simulink model "wheat_line_20_travelling_wind_2019b"  (R2019b)
settings: Solver=FixedStepAuto  StartTime=0.0  StopTime=20  FixedStep=0.001  RelTol=1e-3
values from neighbouring files (symbols this model uses):
  alpha = 50    [run_wheat_line_sway_experiment.m]
  beta = 0    [run_wheat_line_sway_experiment.m]
  edge = 0.1    [natural_freq_experiment.m]    (also in run_wheat_field_sine_wind.m; run_wheat_field_sine_wind_random_height.m; run_wheat_line_experiment.m; run_wheat_line_sway_experiment.m)
  field_length = 4    [natural_freq_experiment.m]    (also in run_wheat_field_sine_wind.m; run_wheat_field_sine_wind_random_height.m; run_wheat_line_experiment.m; run_wheat_line_sway_experiment.m = 8)
  force_amplitude = 5    [natural_freq_experiment.m]    (also in run_wheat_line_sway_experiment.m)
  gain = -800    [natural_freq_experiment.m]    (also in run_wheat_line_experiment.m; run_wheat_line_sway_experiment.m; set_wheat_params.m)
  if_wind_sine = 0    [run_wheat_line_sway_experiment.m]
  wheat_gap = wheat_stem_height/2    (= 0.4)    [natural_freq_experiment.m]    (also in run_wheat_field_sine_wind.m; run_wheat_field_sine_wind_random_height.m; run_wheat_line_experiment.m; run_wheat_line_sway_experiment.m)
  wheat_grain_height = 0.15    [natural_freq_experiment.m]    (also in run_wheat_field_sine_wind.m; run_wheat_field_sine_wind_random_height.m; run_wheat_line_experiment.m; run_wheat_line_sway_experiment.m)
  wheat_grain_radius = 0.03    [natural_freq_experiment.m]    (also in run_wheat_field_sine_wind.m; run_wheat_field_sine_wind_random_height.m; run_wheat_line_experiment.m; run_wheat_line_sway_experiment.m)
  wind_amplitude = 1    [create_travelling_wind_rectangle.m]    (also in create_travelling_wind_sine.m; run_wheat_line_sway_experiment.m)
  wind_frequency = 2    [create_travelling_wind_rectangle.m]    (also in create_travelling_wind_sine.m = 5; run_wheat_line_sway_experiment.m = 50)
  wind_phase_cycle = 5    [create_travelling_wind_rectangle.m]    (also in create_travelling_wind_sine.m = 10; run_wheat_line_sway_experiment.m = 250)
undefined symbols (not defined in the file or in its folder): force_frequency, X, Y, Z
libraries: sm_lib x145, nesl_utility x101, dspmtrx3 x2, dspindex x2, simulink x2
(part 1 of 11)
settings Model: Creator=yz655  LastModifiedBy=Emily

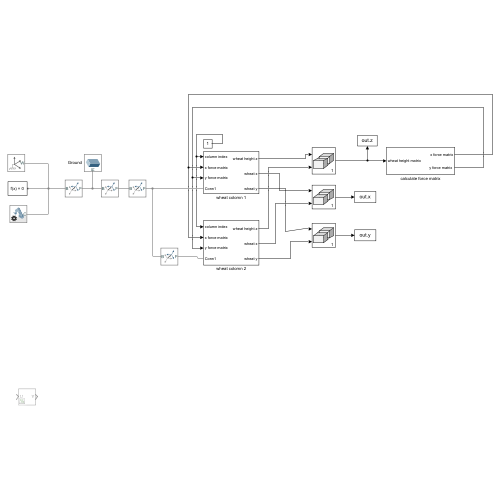
[thumbnail: Simulink's stored preview of the top-level diagram]
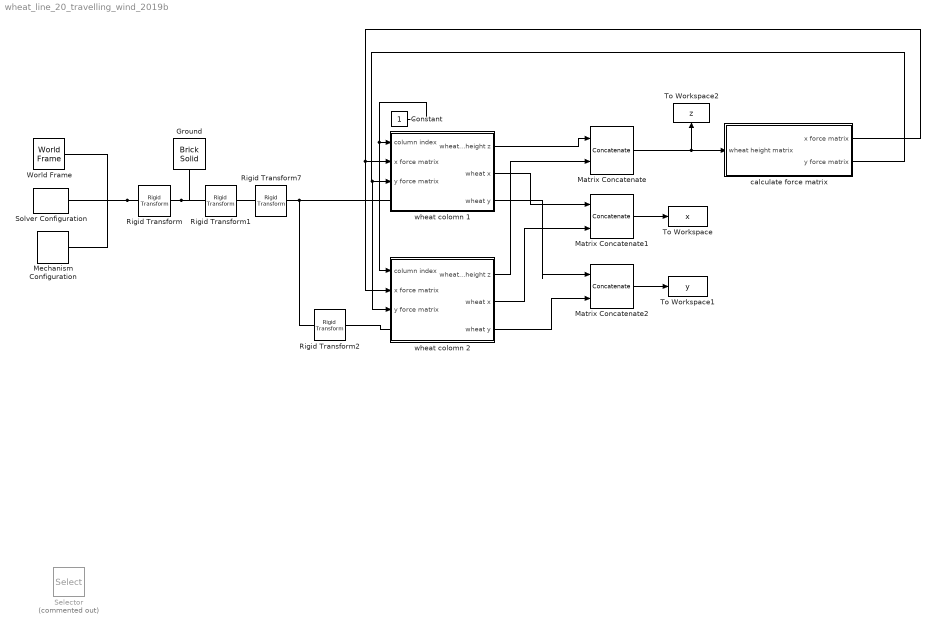
== system wheat_line_20_travelling_wind_2019b ==
  Constant : Constant
  Ground : sm_lib/Body Elements/Brick Solid  GraphicAmbientColor=[0.15 0.15 0.15 1.0]  BasedOnType=Density  BrickDimensions=[field_length 2*field_length 0.1]  BrickDimensionUnits=m  CenterOfMass=[0 0 0]  CenterOfMassUnits=m  GraphicDiffuseColor=[0.5 0.5 0.5]  Density=1000  DensityUnits=kg/m^3  DoExposeReferenceFrame=on  GraphicEmissiveColor=[0.0 0.0 0.0 1.0]  ExportEntireGeometry=off  SerializedFrames=<Frames/>  MarkerShape=Sphere  MarkerSize=10  GraphicType=FromGeometry  InertiaType=CalculateFromGeometry  Mass=1  MassUnits=kg  MomentsOfInertia=[1 1 1]  MomentsOfInertiaUnits=kg*m^2  GraphicOpacity=1.0  ProductsOfInertia=[0 0 0]  ProductsOfInertiaUnits=kg*m^2  GraphicShininess=75  GraphicSpecularColor=[0.5 0.5 0.5 1.0]  GraphicVisPropType=SimpleVisualProperties
  Matrix Concatenate : Concatenate  Mode=Multidimensional array
  Matrix Concatenate1 : Concatenate  Mode=Multidimensional array
  Matrix Concatenate2 : Concatenate  Mode=Multidimensional array
  Mechanism Configuration : sm_lib/Utilities/Mechanism Configuration  UniformGravity=Constant  GravityVector=[0 0 -9.80665]  GravityUnits=m/s^2  LinearizationDelta=0.001  JointModeTransitionNonlinearIterations=2
  Rigid Transform : sm_lib/Frames and Transforms/Rigid Transform  TranslationMethod=None  TranslationStandardOffset=0  TranslationLengthUnit=m  TranslationStandardAxis=+Z  TranslationCartesianOffset=[0 0 0]  TranslationROffset=0  TranslationROffsetUnits=m  TranslationZOffset=0  TranslationZOffsetUnits=m  TranslationThetaOffset=0  TranslationThetaOffsetUnits=deg  RotationMethod=None  RotationAngleUnits=deg  RotationStandardAxis=+Z  RotationAngle=0.0  RotationArbitraryAxis=[0 0 1]  FollAlignAxisA=+X  BaseAlignAxisA=+Y  FollAlignAxisB=+Y  BaseAlignAxisB=+Z  RotationSequenceAxes=FollowerAxes  RotationSequence=XYX  RotationSequenceAngles=[0 0 0]  RotationSequenceAnglesUnits=deg  RotationMatrix=[1 0 0; 0 1 0; 0 0 1]
  Rigid Transform1 : sm_lib/Frames and Transforms/Rigid Transform  TranslationMethod=Cartesian  TranslationStandardOffset=0  TranslationLengthUnit=m  TranslationStandardAxis=+Z  TranslationCartesianOffset=[-field_length/2+edge -field_length+edge 0]  TranslationROffset=0  TranslationROffsetUnits=m  TranslationZOffset=0  TranslationZOffsetUnits=m  TranslationThetaOffset=0  TranslationThetaOffsetUnits=deg  RotationMethod=None  RotationAngleUnits=deg  RotationStandardAxis=+Z  RotationAngle=0.0  RotationArbitraryAxis=[0 0 1]  FollAlignAxisA=+Z  BaseAlignAxisA=+Y  FollAlignAxisB=+Y  BaseAlignAxisB=+Z  RotationSequenceAxes=FollowerAxes  RotationSequence=XYX  RotationSequenceAngles=[0 0 0]  RotationSequenceAnglesUnits=deg  RotationMatrix=[1 0 0; 0 1 0; 0 0 1]
  Rigid Transform2 : sm_lib/Frames and Transforms/Rigid Transform  TranslationMethod=Cartesian  TranslationStandardOffset=0  TranslationLengthUnit=m  TranslationStandardAxis=+Z  TranslationCartesianOffset=[0 10*wheat_gap 0]  TranslationROffset=0  TranslationROffsetUnits=m  TranslationZOffset=0  TranslationZOffsetUnits=m  TranslationThetaOffset=0  TranslationThetaOffsetUnits=deg  RotationMethod=None  RotationAngleUnits=deg  RotationStandardAxis=+Z  RotationAngle=0.0  RotationArbitraryAxis=[0 0 1]  FollAlignAxisA=+Z  BaseAlignAxisA=+Y  FollAlignAxisB=+Y  BaseAlignAxisB=+Z  RotationSequenceAxes=FollowerAxes  RotationSequence=XYX  RotationSequenceAngles=[0 0 0]  RotationSequenceAnglesUnits=deg  RotationMatrix=[1 0 0; 0 1 0; 0 0 1]
  Rigid Transform7 : sm_lib/Frames and Transforms/Rigid Transform  TranslationMethod=Cartesian  TranslationStandardOffset=0  TranslationLengthUnit=m  TranslationStandardAxis=+Z  TranslationCartesianOffset=[0 0 0.05]  TranslationROffset=0  TranslationROffsetUnits=m  TranslationZOffset=0  TranslationZOffsetUnits=m  TranslationThetaOffset=0  TranslationThetaOffsetUnits=deg  RotationMethod=None  RotationAngleUnits=deg  RotationStandardAxis=+Z  RotationAngle=0.0  RotationArbitraryAxis=[0 0 1]  FollAlignAxisA=+Z  BaseAlignAxisA=+Y  FollAlignAxisB=+Y  BaseAlignAxisB=+Z  RotationSequenceAxes=FollowerAxes  RotationSequence=XYX  RotationSequenceAngles=[0 0 0]  RotationSequenceAnglesUnits=deg  RotationMatrix=[1 0 0; 0 1 0; 0 0 1]
  Selector : Selector  Commented=on  NumberOfDimensions=10  InputPortWidth=3  IndexOptions=Index vector (dialog),Index vector (dialog),Index vector (dialog),Index vector (dialog),Index vector (dialog),Index vector (dialog),Index vector (dialog),Index vector (dialog),Index vector (dialog),Index vector (dialog)  Indices=1,1,1,1,1,1,1,1,1,1  OutputSizes=1,1,1,1,1,1,1,1,1,1
  Solver Configuration : nesl_utility/Solver Configuration  PhysicalDomain=network_engine_domain  SubClassName=solver  LeftPortType=input  RightPortType=generic  Tones=[]  Harmonics=[]  SimulateNoise=off  Profile=off  UseLocalSampling=off  EnableSwitchedLinearOptims=on  FrequencyDomain=off  UseCCode=off  RelTol=0.001  AbsTol=1e-06  MinStep=1e-09  ToWorkspace=off  RevertToSquareIcSolve=off  NumHomotopyIterations=100  PhasorMode=off  PhasorModeNumHarmonics=1  DoDC=off  ResidualTolerance=1e-09  UseLocalSolver=off  LocalSolverChoice=NE_BACKWARD_EULER_ADVANCER  LocalSolverSampleTime=0.001  DoFixedCost=off  MaxNonlinIter=3  MaxModeIter=2  ComputeImpulses=off  ImpulseIterations=2  LinearAlgebra=auto  EquationFormulation=NE_TIME_EF  DelaysMemoryBudget=1024  AutomaticFiltering=on  FilteringTimeConstant=0.001  PartitionStorageMethod=AS_NEEDED  PartitionMemoryBudget=1024  PartitionMethod=ROBUST
      settings: SourceProductBaseCode=PW,SS
  To Workspace : ToWorkspace  VariableName=x  SaveFormat=Timeseries  SampleTime=-1
  To Workspace1 : ToWorkspace  VariableName=y  SaveFormat=Timeseries  SampleTime=-1
  To Workspace2 : ToWorkspace  VariableName=z  SaveFormat=Timeseries  SampleTime=-1
  World Frame : sm_lib/Frames and Transforms/World Frame
  "calculate force matrix " : Subsystem
  wheat colomn 1 : Subsystem
  wheat colomn 2 : Subsystem
  wires:
  Matrix Concatenate/1 -> "calculate force matrix "/1(wheat height matrix), To Workspace2/1
  "calculate force matrix "/2("y force matrix ") -> wheat colomn 1/3(y force matrix), wheat colomn 2/3(y force matrix)
  "calculate force matrix "/1(x force matrix) -> wheat colomn 2/2(x force matrix), wheat colomn 1/2(x force matrix)
  Matrix Concatenate1/1 -> To Workspace/1
  wheat colomn 1/3(wheat y) -> Matrix Concatenate2/1
  Matrix Concatenate2/1 -> To Workspace1/1
  wheat colomn 1/2(wheat x) -> Matrix Concatenate1/1
  Constant/1 -> wheat colomn 2/1("column index "), wheat colomn 1/1("column index ")
  wheat colomn 1/1(wheat height z) -> Matrix Concatenate/1
  wheat colomn 2/1(wheat height z) -> Matrix Concatenate/2
  wheat colomn 2/2(wheat x) -> Matrix Concatenate1/2
  wheat colomn 2/3(wheat y) -> Matrix Concatenate2/2
  connections:
  Rigid Transform/LConn1 -- World Frame/RConn1 -- Mechanism Configuration/RConn1 -- Solver Configuration/RConn1
  wheat colomn 1/LConn1 -- Rigid Transform2/LConn1 -- Rigid Transform7/RConn1
  Rigid Transform/RConn1 -- Ground/RConn1 -- Rigid Transform1/LConn1
  Rigid Transform7/LConn1 -- Rigid Transform1/RConn1
  Rigid Transform2/RConn1 -- wheat colomn 2/LConn1

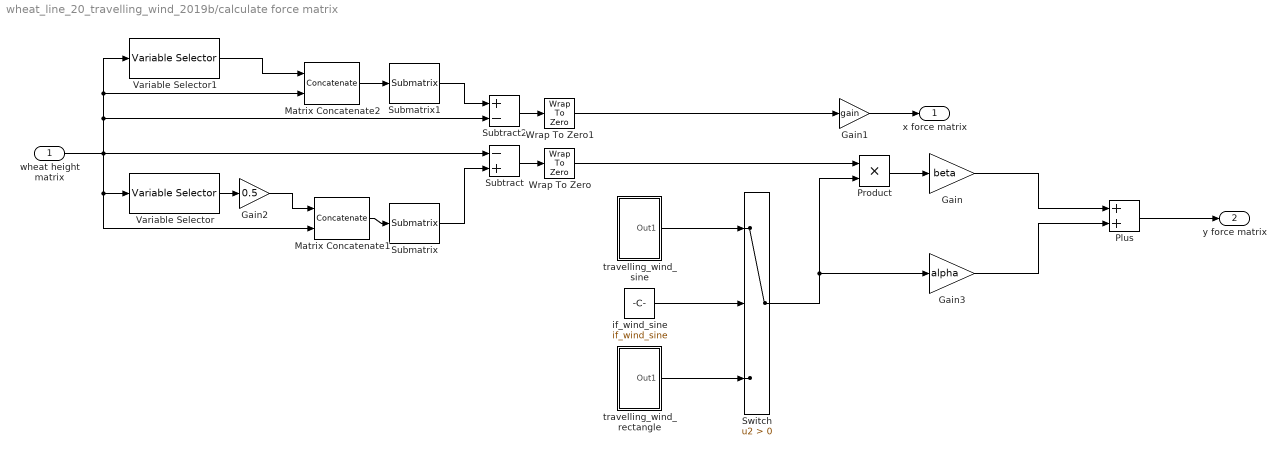
== system wheat_line_20_travelling_wind_2019b/calculate force matrix  ==
  wheat height matrix : Inport
  Gain : Gain  Gain=beta
  Gain1 : Gain  Gain=gain
  Gain2 : Gain  Gain=0.5
  Gain3 : Gain  Gain=alpha
  Matrix Concatenate1 : Concatenate  Mode=Multidimensional array
  Matrix Concatenate2 : Concatenate  Mode=Multidimensional array  ConcatenateDimension=2
  Plus : Sum
  Product : Product
  Submatrix : dspmtrx3/Submatrix  RowSpan=Range of rows  RowStartMode=First  RowStartIndex=1  RowEndMode=Offset from last  RowEndIndex=1  ColSpan=Range of columns  ColStartMode=First  ColStartIndex=1  ColEndMode=Last  ColEndIndex=1
  Submatrix1 : dspmtrx3/Submatrix  RowSpan=Range of rows  RowStartMode=First  RowStartIndex=1  RowEndMode=Last  RowEndIndex=1  ColSpan=Range of columns  ColStartMode=First  ColStartIndex=1  ColEndMode=Offset from last  ColEndIndex=1
  Subtract : Sum  Inputs=-+
  Subtract2 : Sum  Inputs=+-
  Switch : Switch  Criteria=u2 > Threshold
  Variable Selector : dspindex/Variable Selector  NumInputs=1  rowsOrCols=Rows  IdxMode=Fixed  Elements=[1]  ZerOneIdxMode=One-based  errmode=Clip Index  FillMode=on  FillValues=0
  Variable Selector1 : dspindex/Variable Selector  NumInputs=1  rowsOrCols=Columns  IdxMode=Fixed  Elements=[1]  ZerOneIdxMode=One-based  errmode=Clip Index  FillMode=on  FillValues=0
  Wrap To Zero : simulink/Discontinuities/Wrap To Zero  Threshold=0
      settings: SourceProductBaseCode=SL
  Wrap To Zero1 : simulink/Discontinuities/Wrap To Zero  Threshold=0
      settings: SourceProductBaseCode=SL
  if_wind_sine : Constant  Value=if_wind_sine
  travelling_wind_rectangle : Subsystem
  travelling_wind_sine : Subsystem
  x force matrix : Outport
  "y force matrix " : Outport  Port=2
  wires:
  wheat height matrix/1 -> Matrix Concatenate1/2, Variable Selector/1, Variable Selector1/1, Matrix Concatenate2/2, Subtract2/2, Subtract/1
  Submatrix/1 -> Subtract/2
  Variable Selector1/1 -> Matrix Concatenate2/1
  Subtract2/1 -> Wrap To Zero1/1
  Submatrix1/1 -> Subtract2/1
  Matrix Concatenate2/1 -> Submatrix1/1
  Subtract/1 -> Wrap To Zero/1
  Matrix Concatenate1/1 -> Submatrix/1
  Gain1/1 -> x force matrix/1
  Wrap To Zero1/1 -> Gain1/1
  Wrap To Zero/1 -> Product/1
  Product/1 -> Gain/1
  Variable Selector/1 -> Gain2/1
  Gain2/1 -> Matrix Concatenate1/1
  Switch/1 -> Gain3/1, Product/2
  travelling_wind_sine/1(Out1) -> Switch/1
  if_wind_sine/1 -> Switch/2
  travelling_wind_rectangle/1(Out1) -> Switch/3
  Gain/1 -> Plus/1
  Plus/1 -> "y force matrix "/1
  Gain3/1 -> Plus/2

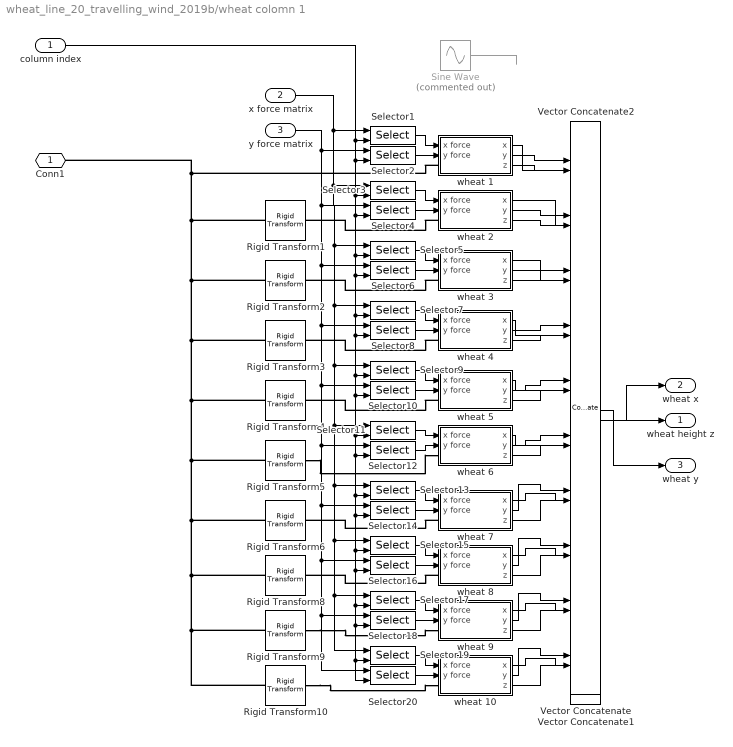
== system wheat_line_20_travelling_wind_2019b/wheat colomn 1 ==
  "column index " : Inport
  x force matrix : Inport  Port=2
  y force matrix : Inport  Port=3
  Rigid Transform1 : sm_lib/Frames and Transforms/Rigid Transform  TranslationMethod=Cartesian  TranslationStandardOffset=0  TranslationLengthUnit=m  TranslationStandardAxis=+Z  TranslationCartesianOffset=[0 wheat_gap 0]  TranslationROffset=0  TranslationROffsetUnits=m  TranslationZOffset=0  TranslationZOffsetUnits=m  TranslationThetaOffset=0  TranslationThetaOffsetUnits=deg  RotationMethod=None  RotationAngleUnits=deg  RotationStandardAxis=+Z  RotationAngle=0.0  RotationArbitraryAxis=[0 0 1]  FollAlignAxisA=+X  BaseAlignAxisA=+Y  FollAlignAxisB=+Y  BaseAlignAxisB=+Z  RotationSequenceAxes=FollowerAxes  RotationSequence=XYX  RotationSequenceAngles=[0 0 0]  RotationSequenceAnglesUnits=deg  RotationMatrix=[1 0 0; 0 1 0; 0 0 1]
  Rigid Transform10 : sm_lib/Frames and Transforms/Rigid Transform  TranslationMethod=Cartesian  TranslationStandardOffset=0  TranslationLengthUnit=m  TranslationStandardAxis=+Z  TranslationCartesianOffset=[0 9*wheat_gap 0]  TranslationROffset=0  TranslationROffsetUnits=m  TranslationZOffset=0  TranslationZOffsetUnits=m  TranslationThetaOffset=0  TranslationThetaOffsetUnits=deg  RotationMethod=None  RotationAngleUnits=deg  RotationStandardAxis=+Z  RotationAngle=0.0  RotationArbitraryAxis=[0 0 1]  FollAlignAxisA=+X  BaseAlignAxisA=+Y  FollAlignAxisB=+Y  BaseAlignAxisB=+Z  RotationSequenceAxes=FollowerAxes  RotationSequence=XYX  RotationSequenceAngles=[0 0 0]  RotationSequenceAnglesUnits=deg  RotationMatrix=[1 0 0; 0 1 0; 0 0 1]
  Rigid Transform2 : sm_lib/Frames and Transforms/Rigid Transform  TranslationMethod=Cartesian  TranslationStandardOffset=0  TranslationLengthUnit=m  TranslationStandardAxis=+Z  TranslationCartesianOffset=[0 2*wheat_gap 0]  TranslationROffset=0  TranslationROffsetUnits=m  TranslationZOffset=0  TranslationZOffsetUnits=m  TranslationThetaOffset=0  TranslationThetaOffsetUnits=deg  RotationMethod=None  RotationAngleUnits=deg  RotationStandardAxis=+Z  RotationAngle=0.0  RotationArbitraryAxis=[0 0 1]  FollAlignAxisA=+X  BaseAlignAxisA=+Y  FollAlignAxisB=+Y  BaseAlignAxisB=+Z  RotationSequenceAxes=FollowerAxes  RotationSequence=XYX  RotationSequenceAngles=[0 0 0]  RotationSequenceAnglesUnits=deg  RotationMatrix=[1 0 0; 0 1 0; 0 0 1]
  Rigid Transform3 : sm_lib/Frames and Transforms/Rigid Transform  TranslationMethod=Cartesian  TranslationStandardOffset=0  TranslationLengthUnit=m  TranslationStandardAxis=+Z  TranslationCartesianOffset=[0 3*wheat_gap 0]  TranslationROffset=0  TranslationROffsetUnits=m  TranslationZOffset=0  TranslationZOffsetUnits=m  TranslationThetaOffset=0  TranslationThetaOffsetUnits=deg  RotationMethod=None  RotationAngleUnits=deg  RotationStandardAxis=+Z  RotationAngle=0.0  RotationArbitraryAxis=[0 0 1]  FollAlignAxisA=+X  BaseAlignAxisA=+Y  FollAlignAxisB=+Y  BaseAlignAxisB=+Z  RotationSequenceAxes=FollowerAxes  RotationSequence=XYX  RotationSequenceAngles=[0 0 0]  RotationSequenceAnglesUnits=deg  RotationMatrix=[1 0 0; 0 1 0; 0 0 1]
  Rigid Transform4 : sm_lib/Frames and Transforms/Rigid Transform  TranslationMethod=Cartesian  TranslationStandardOffset=0  TranslationLengthUnit=m  TranslationStandardAxis=+Z  TranslationCartesianOffset=[0 4*wheat_gap 0]  TranslationROffset=0  TranslationROffsetUnits=m  TranslationZOffset=0  TranslationZOffsetUnits=m  TranslationThetaOffset=0  TranslationThetaOffsetUnits=deg  RotationMethod=None  RotationAngleUnits=deg  RotationStandardAxis=+Z  RotationAngle=0.0  RotationArbitraryAxis=[0 0 1]  FollAlignAxisA=+X  BaseAlignAxisA=+Y  FollAlignAxisB=+Y  BaseAlignAxisB=+Z  RotationSequenceAxes=FollowerAxes  RotationSequence=XYX  RotationSequenceAngles=[0 0 0]  RotationSequenceAnglesUnits=deg  RotationMatrix=[1 0 0; 0 1 0; 0 0 1]
  Rigid Transform5 : sm_lib/Frames and Transforms/Rigid Transform  TranslationMethod=Cartesian  TranslationStandardOffset=0  TranslationLengthUnit=m  TranslationStandardAxis=+Z  TranslationCartesianOffset=[0 5*wheat_gap 0]  TranslationROffset=0  TranslationROffsetUnits=m  TranslationZOffset=0  TranslationZOffsetUnits=m  TranslationThetaOffset=0  TranslationThetaOffsetUnits=deg  RotationMethod=None  RotationAngleUnits=deg  RotationStandardAxis=+Z  RotationAngle=0.0  RotationArbitraryAxis=[0 0 1]  FollAlignAxisA=+X  BaseAlignAxisA=+Y  FollAlignAxisB=+Y  BaseAlignAxisB=+Z  RotationSequenceAxes=FollowerAxes  RotationSequence=XYX  RotationSequenceAngles=[0 0 0]  RotationSequenceAnglesUnits=deg  RotationMatrix=[1 0 0; 0 1 0; 0 0 1]
  Rigid Transform6 : sm_lib/Frames and Transforms/Rigid Transform  TranslationMethod=Cartesian  TranslationStandardOffset=0  TranslationLengthUnit=m  TranslationStandardAxis=+Z  TranslationCartesianOffset=[0 6*wheat_gap 0]  TranslationROffset=0  TranslationROffsetUnits=m  TranslationZOffset=0  TranslationZOffsetUnits=m  TranslationThetaOffset=0  TranslationThetaOffsetUnits=deg  RotationMethod=None  RotationAngleUnits=deg  RotationStandardAxis=+Z  RotationAngle=0.0  RotationArbitraryAxis=[0 0 1]  FollAlignAxisA=+X  BaseAlignAxisA=+Y  FollAlignAxisB=+Y  BaseAlignAxisB=+Z  RotationSequenceAxes=FollowerAxes  RotationSequence=XYX  RotationSequenceAngles=[0 0 0]  RotationSequenceAnglesUnits=deg  RotationMatrix=[1 0 0; 0 1 0; 0 0 1]
  Rigid Transform8 : sm_lib/Frames and Transforms/Rigid Transform  TranslationMethod=Cartesian  TranslationStandardOffset=0  TranslationLengthUnit=m  TranslationStandardAxis=+Z  TranslationCartesianOffset=[0 7*wheat_gap 0]  TranslationROffset=0  TranslationROffsetUnits=m  TranslationZOffset=0  TranslationZOffsetUnits=m  TranslationThetaOffset=0  TranslationThetaOffsetUnits=deg  RotationMethod=None  RotationAngleUnits=deg  RotationStandardAxis=+Z  RotationAngle=0.0  RotationArbitraryAxis=[0 0 1]  FollAlignAxisA=+X  BaseAlignAxisA=+Y  FollAlignAxisB=+Y  BaseAlignAxisB=+Z  RotationSequenceAxes=FollowerAxes  RotationSequence=XYX  RotationSequenceAngles=[0 0 0]  RotationSequenceAnglesUnits=deg  RotationMatrix=[1 0 0; 0 1 0; 0 0 1]
  Rigid Transform9 : sm_lib/Frames and Transforms/Rigid Transform  TranslationMethod=Cartesian  TranslationStandardOffset=0  TranslationLengthUnit=m  TranslationStandardAxis=+Z  TranslationCartesianOffset=[0 8*wheat_gap 0]  TranslationROffset=0  TranslationROffsetUnits=m  TranslationZOffset=0  TranslationZOffsetUnits=m  TranslationThetaOffset=0  TranslationThetaOffsetUnits=deg  RotationMethod=None  RotationAngleUnits=deg  RotationStandardAxis=+Z  RotationAngle=0.0  RotationArbitraryAxis=[0 0 1]  FollAlignAxisA=+X  BaseAlignAxisA=+Y  FollAlignAxisB=+Y  BaseAlignAxisB=+Z  RotationSequenceAxes=FollowerAxes  RotationSequence=XYX  RotationSequenceAngles=[0 0 0]  RotationSequenceAnglesUnits=deg  RotationMatrix=[1 0 0; 0 1 0; 0 0 1]
  Selector1 : Selector  NumberOfDimensions=2  InputPortWidth=3  IndexOptions=Index vector (dialog),Index vector (port)  Indices=1,1  OutputSizes=1,1
  Selector10 : Selector  NumberOfDimensions=2  InputPortWidth=3  IndexOptions=Index vector (dialog),Index vector (port)  Indices=5,1  OutputSizes=1,1
  Selector11 : Selector  NumberOfDimensions=2  InputPortWidth=3  IndexOptions=Index vector (dialog),Index vector (port)  Indices=6,1  OutputSizes=1,1
  Selector12 : Selector  NumberOfDimensions=2  InputPortWidth=3  IndexOptions=Index vector (dialog),Index vector (port)  Indices=6,1  OutputSizes=1,1
  Selector13 : Selector  NumberOfDimensions=2  InputPortWidth=3  IndexOptions=Index vector (dialog),Index vector (port)  Indices=7,1  OutputSizes=1,1
  Selector14 : Selector  NumberOfDimensions=2  InputPortWidth=3  IndexOptions=Index vector (dialog),Index vector (port)  Indices=7,1  OutputSizes=1,1
  Selector15 : Selector  NumberOfDimensions=2  InputPortWidth=3  IndexOptions=Index vector (dialog),Index vector (port)  Indices=8,1  OutputSizes=1,1
  Selector16 : Selector  NumberOfDimensions=2  InputPortWidth=3  IndexOptions=Index vector (dialog),Index vector (port)  Indices=8,1  OutputSizes=1,1
  Selector17 : Selector  NumberOfDimensions=2  InputPortWidth=3  IndexOptions=Index vector (dialog),Index vector (port)  Indices=9,1  OutputSizes=1,1
  Selector18 : Selector  NumberOfDimensions=2  InputPortWidth=3  IndexOptions=Index vector (dialog),Index vector (port)  Indices=9,1  OutputSizes=1,1
  Selector19 : Selector  NumberOfDimensions=2  InputPortWidth=3  IndexOptions=Index vector (dialog),Index vector (port)  Indices=10,1  OutputSizes=1,1
  Selector2 : Selector  NumberOfDimensions=2  InputPortWidth=3  IndexOptions=Index vector (dialog),Index vector (port)  Indices=1,1  OutputSizes=1,1
  Selector20 : Selector  NumberOfDimensions=2  InputPortWidth=3  IndexOptions=Index vector (dialog),Index vector (port)  Indices=10,1  OutputSizes=1,1
  Selector3 : Selector  NumberOfDimensions=2  InputPortWidth=3  IndexOptions=Index vector (dialog),Index vector (port)  Indices=2,1  OutputSizes=1,1
  Selector4 : Selector  NumberOfDimensions=2  InputPortWidth=3  IndexOptions=Index vector (dialog),Index vector (port)  Indices=2,1  OutputSizes=1,1
  Selector5 : Selector  NumberOfDimensions=2  InputPortWidth=3  IndexOptions=Index vector (dialog),Index vector (port)  Indices=3,1  OutputSizes=1,1
  Selector6 : Selector  NumberOfDimensions=2  InputPortWidth=3  IndexOptions=Index vector (dialog),Index vector (port)  Indices=3,1  OutputSizes=1,1
  Selector7 : Selector  NumberOfDimensions=2  InputPortWidth=3  IndexOptions=Index vector (dialog),Index vector (port)  Indices=4,1  OutputSizes=1,1
  Selector8 : Selector  NumberOfDimensions=2  InputPortWidth=3  IndexOptions=Index vector (dialog),Index vector (port)  Indices=4,1  OutputSizes=1,1
  Selector9 : Selector  NumberOfDimensions=2  InputPortWidth=3  IndexOptions=Index vector (dialog),Index vector (port)  Indices=5,1  OutputSizes=1,1
  Sine Wave : Sin  Commented=on  Amplitude=force_amplitude  Frequency=force_frequency  SampleTime=0
  Vector Concatenate : Concatenate  NumInputs=10
  Vector Concatenate1 : Concatenate  NumInputs=10
  Vector Concatenate2 : Concatenate  NumInputs=10
  wheat 1 : Subsystem
  wheat 10 : Subsystem
  wheat 2 : Subsystem
  wheat 3 : Subsystem
  wheat 4 : Subsystem
  wheat 5 : Subsystem
  wheat 6 : Subsystem
  wheat 7 : Subsystem
  wheat 8 : Subsystem
  wheat 9 : Subsystem
  Conn1 : PMIOPort  Side=Left
  wheat height z : Outport
  wheat x : Outport  Port=2
  wheat y : Outport  Port=3
  wires:
  Vector Concatenate/1 -> wheat height z/1
  x force matrix/1 -> Selector1/1, Selector3/1, Selector19/1, Selector17/1, Selector15/1, Selector13/1, Selector11/1, Selector9/1, Selector7/1, Selector5/1
  "column index "/1 -> Selector20/2, Selector19/2, Selector18/2, Selector17/2, Selector16/2, Selector15/2, Selector14/2, Selector13/2, Selector12/2, Selector11/2, Selector10/2, Selector9/2, Selector8/2, Selector7/2, Selector6/2, Selector5/2, Selector4/2, Selector3/2, Selector2/2, Selector1/2
  wheat 1/3(z) -> Vector Concatenate/1
  wheat 9/3(z) -> Vector Concatenate/9
  Selector1/1 -> wheat 1/1(x force)
  Selector13/1 -> wheat 7/1(x force)
  Selector5/1 -> wheat 3/1(x force)
  Selector19/1 -> wheat 10/1(x force)
  Selector16/1 -> wheat 8/2(y force)
  Selector9/1 -> wheat 5/1(x force)
  Selector6/1 -> wheat 3/2(y force)
  Selector15/1 -> wheat 8/1(x force)
  Selector7/1 -> wheat 4/1(x force)
  Selector14/1 -> wheat 7/2(y force)
  Selector11/1 -> wheat 6/1(x force)
  Selector8/1 -> wheat 4/2(y force)
  Selector4/1 -> wheat 2/2(y force)
  Selector20/1 -> wheat 10/2(y force)
  Selector2/1 -> wheat 1/2(y force)
  Selector10/1 -> wheat 5/2(y force)
  wheat 6/3(z) -> Vector Concatenate/6
  Selector12/1 -> wheat 6/2(y force)
  Selector3/1 -> wheat 2/1(x force)
  wheat 10/3(z) -> Vector Concatenate/10
  Selector17/1 -> wheat 9/1(x force)
  y force matrix/1 -> Selector2/1, Selector8/1, Selector20/1, Selector18/1, Selector16/1, Selector14/1, Selector12/1, Selector10/1, Selector6/1, Selector4/1
  Selector18/1 -> wheat 9/2(y force)
  wheat 8/3(z) -> Vector Concatenate/8
  wheat 7/3(z) -> Vector Concatenate/7
  wheat 5/3(z) -> Vector Concatenate/5
  wheat 3/3(z) -> Vector Concatenate/3
  wheat 2/3(z) -> Vector Concatenate/2
  wheat 4/3(z) -> Vector Concatenate/4
  wheat 2/1(x) -> Vector Concatenate1/2
  wheat 3/1(x) -> Vector Concatenate1/3
  wheat 4/1(x) -> Vector Concatenate1/4
  wheat 9/1(x) -> Vector Concatenate1/9
  wheat 10/1(x) -> Vector Concatenate1/10
  Vector Concatenate1/1 -> wheat x/1
  wheat 7/1(x) -> Vector Concatenate1/7
  wheat 5/1(x) -> Vector Concatenate1/5
  wheat 6/1(x) -> Vector Concatenate1/6
  wheat 8/1(x) -> Vector Concatenate1/8
  wheat 1/1(x) -> Vector Concatenate1/1
  wheat 2/2(y) -> Vector Concatenate2/2
  wheat 3/2(y) -> Vector Concatenate2/3
  wheat 4/2(y) -> Vector Concatenate2/4
  wheat 9/2(y) -> Vector Concatenate2/9
  wheat 10/2(y) -> Vector Concatenate2/10
  Vector Concatenate2/1 -> wheat y/1
  wheat 7/2(y) -> Vector Concatenate2/7
  wheat 5/2(y) -> Vector Concatenate2/5
  wheat 6/2(y) -> Vector Concatenate2/6
  wheat 8/2(y) -> Vector Concatenate2/8
  wheat 1/2(y) -> Vector Concatenate2/1
  Sine Wave/1 -> ?
  connections:
  wheat 5/LConn1 -- Rigid Transform4/RConn1
  wheat 3/LConn1 -- Rigid Transform2/RConn1
  wheat 4/LConn1 -- Rigid Transform3/RConn1
  Rigid Transform5/RConn1 -- wheat 6/LConn1
  Rigid Transform9/RConn1 -- wheat 9/LConn1
  wheat 8/LConn1 -- Rigid Transform8/RConn1
  wheat 7/LConn1 -- Rigid Transform6/RConn1
  Rigid Transform10/RConn1 -- wheat 10/LConn1
  wheat 2/LConn1 -- Rigid Transform1/RConn1
  Rigid Transform10/LConn1 -- Rigid Transform9/LConn1 -- Rigid Transform8/LConn1 -- Rigid Transform6/LConn1 -- Rigid Transform5/LConn1 -- Rigid Transform4/LConn1 -- Rigid Transform3/LConn1 -- Rigid Transform2/LConn1 -- Rigid Transform1/LConn1 -- Conn1/RConn1 -- wheat 1/LConn1

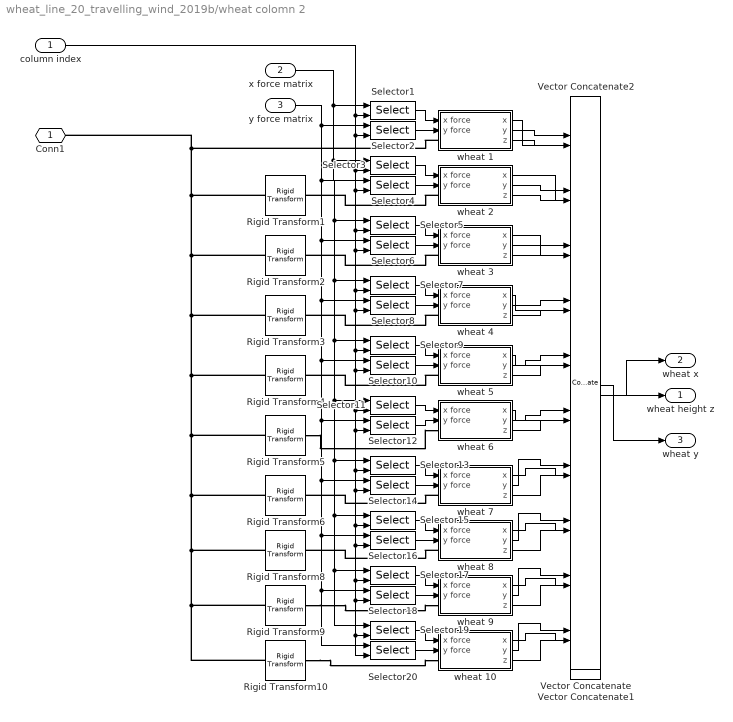
== system wheat_line_20_travelling_wind_2019b/wheat colomn 2 ==
  "column index " : Inport
  x force matrix : Inport  Port=2
  y force matrix : Inport  Port=3
  Rigid Transform1 : sm_lib/Frames and Transforms/Rigid Transform  TranslationMethod=Cartesian  TranslationStandardOffset=0  TranslationLengthUnit=m  TranslationStandardAxis=+Z  TranslationCartesianOffset=[0 wheat_gap 0]  TranslationROffset=0  TranslationROffsetUnits=m  TranslationZOffset=0  TranslationZOffsetUnits=m  TranslationThetaOffset=0  TranslationThetaOffsetUnits=deg  RotationMethod=None  RotationAngleUnits=deg  RotationStandardAxis=+Z  RotationAngle=0.0  RotationArbitraryAxis=[0 0 1]  FollAlignAxisA=+X  BaseAlignAxisA=+Y  FollAlignAxisB=+Y  BaseAlignAxisB=+Z  RotationSequenceAxes=FollowerAxes  RotationSequence=XYX  RotationSequenceAngles=[0 0 0]  RotationSequenceAnglesUnits=deg  RotationMatrix=[1 0 0; 0 1 0; 0 0 1]
  Rigid Transform10 : sm_lib/Frames and Transforms/Rigid Transform  TranslationMethod=Cartesian  TranslationStandardOffset=0  TranslationLengthUnit=m  TranslationStandardAxis=+Z  TranslationCartesianOffset=[0 9*wheat_gap 0]  TranslationROffset=0  TranslationROffsetUnits=m  TranslationZOffset=0  TranslationZOffsetUnits=m  TranslationThetaOffset=0  TranslationThetaOffsetUnits=deg  RotationMethod=None  RotationAngleUnits=deg  RotationStandardAxis=+Z  RotationAngle=0.0  RotationArbitraryAxis=[0 0 1]  FollAlignAxisA=+X  BaseAlignAxisA=+Y  FollAlignAxisB=+Y  BaseAlignAxisB=+Z  RotationSequenceAxes=FollowerAxes  RotationSequence=XYX  RotationSequenceAngles=[0 0 0]  RotationSequenceAnglesUnits=deg  RotationMatrix=[1 0 0; 0 1 0; 0 0 1]
  Rigid Transform2 : sm_lib/Frames and Transforms/Rigid Transform  TranslationMethod=Cartesian  TranslationStandardOffset=0  TranslationLengthUnit=m  TranslationStandardAxis=+Z  TranslationCartesianOffset=[0 2*wheat_gap 0]  TranslationROffset=0  TranslationROffsetUnits=m  TranslationZOffset=0  TranslationZOffsetUnits=m  TranslationThetaOffset=0  TranslationThetaOffsetUnits=deg  RotationMethod=None  RotationAngleUnits=deg  RotationStandardAxis=+Z  RotationAngle=0.0  RotationArbitraryAxis=[0 0 1]  FollAlignAxisA=+X  BaseAlignAxisA=+Y  FollAlignAxisB=+Y  BaseAlignAxisB=+Z  RotationSequenceAxes=FollowerAxes  RotationSequence=XYX  RotationSequenceAngles=[0 0 0]  RotationSequenceAnglesUnits=deg  RotationMatrix=[1 0 0; 0 1 0; 0 0 1]
  Rigid Transform3 : sm_lib/Frames and Transforms/Rigid Transform  TranslationMethod=Cartesian  TranslationStandardOffset=0  TranslationLengthUnit=m  TranslationStandardAxis=+Z  TranslationCartesianOffset=[0 3*wheat_gap 0]  TranslationROffset=0  TranslationROffsetUnits=m  TranslationZOffset=0  TranslationZOffsetUnits=m  TranslationThetaOffset=0  TranslationThetaOffsetUnits=deg  RotationMethod=None  RotationAngleUnits=deg  RotationStandardAxis=+Z  RotationAngle=0.0  RotationArbitraryAxis=[0 0 1]  FollAlignAxisA=+X  BaseAlignAxisA=+Y  FollAlignAxisB=+Y  BaseAlignAxisB=+Z  RotationSequenceAxes=FollowerAxes  RotationSequence=XYX  RotationSequenceAngles=[0 0 0]  RotationSequenceAnglesUnits=deg  RotationMatrix=[1 0 0; 0 1 0; 0 0 1]
  Rigid Transform4 : sm_lib/Frames and Transforms/Rigid Transform  TranslationMethod=Cartesian  TranslationStandardOffset=0  TranslationLengthUnit=m  TranslationStandardAxis=+Z  TranslationCartesianOffset=[0 4*wheat_gap 0]  TranslationROffset=0  TranslationROffsetUnits=m  TranslationZOffset=0  TranslationZOffsetUnits=m  TranslationThetaOffset=0  TranslationThetaOffsetUnits=deg  RotationMethod=None  RotationAngleUnits=deg  RotationStandardAxis=+Z  RotationAngle=0.0  RotationArbitraryAxis=[0 0 1]  FollAlignAxisA=+X  BaseAlignAxisA=+Y  FollAlignAxisB=+Y  BaseAlignAxisB=+Z  RotationSequenceAxes=FollowerAxes  RotationSequence=XYX  RotationSequenceAngles=[0 0 0]  RotationSequenceAnglesUnits=deg  RotationMatrix=[1 0 0; 0 1 0; 0 0 1]
  Rigid Transform5 : sm_lib/Frames and Transforms/Rigid Transform  TranslationMethod=Cartesian  TranslationStandardOffset=0  TranslationLengthUnit=m  TranslationStandardAxis=+Z  TranslationCartesianOffset=[0 5*wheat_gap 0]  TranslationROffset=0  TranslationROffsetUnits=m  TranslationZOffset=0  TranslationZOffsetUnits=m  TranslationThetaOffset=0  TranslationThetaOffsetUnits=deg  RotationMethod=None  RotationAngleUnits=deg  RotationStandardAxis=+Z  RotationAngle=0.0  RotationArbitraryAxis=[0 0 1]  FollAlignAxisA=+X  BaseAlignAxisA=+Y  FollAlignAxisB=+Y  BaseAlignAxisB=+Z  RotationSequenceAxes=FollowerAxes  RotationSequence=XYX  RotationSequenceAngles=[0 0 0]  RotationSequenceAnglesUnits=deg  RotationMatrix=[1 0 0; 0 1 0; 0 0 1]
  Rigid Transform6 : sm_lib/Frames and Transforms/Rigid Transform  TranslationMethod=Cartesian  TranslationStandardOffset=0  TranslationLengthUnit=m  TranslationStandardAxis=+Z  TranslationCartesianOffset=[0 6*wheat_gap 0]  TranslationROffset=0  TranslationROffsetUnits=m  TranslationZOffset=0  TranslationZOffsetUnits=m  TranslationThetaOffset=0  TranslationThetaOffsetUnits=deg  RotationMethod=None  RotationAngleUnits=deg  RotationStandardAxis=+Z  RotationAngle=0.0  RotationArbitraryAxis=[0 0 1]  FollAlignAxisA=+X  BaseAlignAxisA=+Y  FollAlignAxisB=+Y  BaseAlignAxisB=+Z  RotationSequenceAxes=FollowerAxes  RotationSequence=XYX  RotationSequenceAngles=[0 0 0]  RotationSequenceAnglesUnits=deg  RotationMatrix=[1 0 0; 0 1 0; 0 0 1]
  Rigid Transform8 : sm_lib/Frames and Transforms/Rigid Transform  TranslationMethod=Cartesian  TranslationStandardOffset=0  TranslationLengthUnit=m  TranslationStandardAxis=+Z  TranslationCartesianOffset=[0 7*wheat_gap 0]  TranslationROffset=0  TranslationROffsetUnits=m  TranslationZOffset=0  TranslationZOffsetUnits=m  TranslationThetaOffset=0  TranslationThetaOffsetUnits=deg  RotationMethod=None  RotationAngleUnits=deg  RotationStandardAxis=+Z  RotationAngle=0.0  RotationArbitraryAxis=[0 0 1]  FollAlignAxisA=+X  BaseAlignAxisA=+Y  FollAlignAxisB=+Y  BaseAlignAxisB=+Z  RotationSequenceAxes=FollowerAxes  RotationSequence=XYX  RotationSequenceAngles=[0 0 0]  RotationSequenceAnglesUnits=deg  RotationMatrix=[1 0 0; 0 1 0; 0 0 1]
  Rigid Transform9 : sm_lib/Frames and Transforms/Rigid Transform  TranslationMethod=Cartesian  TranslationStandardOffset=0  TranslationLengthUnit=m  TranslationStandardAxis=+Z  TranslationCartesianOffset=[0 8*wheat_gap 0]  TranslationROffset=0  TranslationROffsetUnits=m  TranslationZOffset=0  TranslationZOffsetUnits=m  TranslationThetaOffset=0  TranslationThetaOffsetUnits=deg  RotationMethod=None  RotationAngleUnits=deg  RotationStandardAxis=+Z  RotationAngle=0.0  RotationArbitraryAxis=[0 0 1]  FollAlignAxisA=+X  BaseAlignAxisA=+Y  FollAlignAxisB=+Y  BaseAlignAxisB=+Z  RotationSequenceAxes=FollowerAxes  RotationSequence=XYX  RotationSequenceAngles=[0 0 0]  RotationSequenceAnglesUnits=deg  RotationMatrix=[1 0 0; 0 1 0; 0 0 1]
  Selector1 : Selector  NumberOfDimensions=2  InputPortWidth=3  IndexOptions=Index vector (dialog),Index vector (port)  Indices=1,11  OutputSizes=1,1
  Selector10 : Selector  NumberOfDimensions=2  InputPortWidth=3  IndexOptions=Index vector (dialog),Index vector (port)  Indices=15,1  OutputSizes=1,1
  Selector11 : Selector  NumberOfDimensions=2  InputPortWidth=3  IndexOptions=Index vector (dialog),Index vector (port)  Indices=16,1  OutputSizes=1,1
  Selector12 : Selector  NumberOfDimensions=2  InputPortWidth=3  IndexOptions=Index vector (dialog),Index vector (port)  Indices=16,1  OutputSizes=1,1
  Selector13 : Selector  NumberOfDimensions=2  InputPortWidth=3  IndexOptions=Index vector (dialog),Index vector (port)  Indices=17,1  OutputSizes=1,1
  Selector14 : Selector  NumberOfDimensions=2  InputPortWidth=3  IndexOptions=Index vector (dialog),Index vector (port)  Indices=17,1  OutputSizes=1,1
  Selector15 : Selector  NumberOfDimensions=2  InputPortWidth=3  IndexOptions=Index vector (dialog),Index vector (port)  Indices=18,1  OutputSizes=1,1
  Selector16 : Selector  NumberOfDimensions=2  InputPortWidth=3  IndexOptions=Index vector (dialog),Index vector (port)  Indices=18,1  OutputSizes=1,1
  Selector17 : Selector  NumberOfDimensions=2  InputPortWidth=3  IndexOptions=Index vector (dialog),Index vector (port)  Indices=19,1  OutputSizes=1,1
  Selector18 : Selector  NumberOfDimensions=2  InputPortWidth=3  IndexOptions=Index vector (dialog),Index vector (port)  Indices=19,1  OutputSizes=1,1
  Selector19 : Selector  NumberOfDimensions=2  InputPortWidth=3  IndexOptions=Index vector (dialog),Index vector (port)  Indices=20,1  OutputSizes=1,1
  Selector2 : Selector  NumberOfDimensions=2  InputPortWidth=3  IndexOptions=Index vector (dialog),Index vector (port)  Indices=11,1  OutputSizes=1,1
  Selector20 : Selector  NumberOfDimensions=2  InputPortWidth=3  IndexOptions=Index vector (dialog),Index vector (port)  Indices=20,1  OutputSizes=1,1
  Selector3 : Selector  NumberOfDimensions=2  InputPortWidth=3  IndexOptions=Index vector (dialog),Index vector (port)  Indices=12,1  OutputSizes=1,1
  Selector4 : Selector  NumberOfDimensions=2  InputPortWidth=3  IndexOptions=Index vector (dialog),Index vector (port)  Indices=12,1  OutputSizes=1,1
  Selector5 : Selector  NumberOfDimensions=2  InputPortWidth=3  IndexOptions=Index vector (dialog),Index vector (port)  Indices=13,1  OutputSizes=1,1
  Selector6 : Selector  NumberOfDimensions=2  InputPortWidth=3  IndexOptions=Index vector (dialog),Index vector (port)  Indices=13,1  OutputSizes=1,1
  Selector7 : Selector  NumberOfDimensions=2  InputPortWidth=3  IndexOptions=Index vector (dialog),Index vector (port)  Indices=14,1  OutputSizes=1,1
  Selector8 : Selector  NumberOfDimensions=2  InputPortWidth=3  IndexOptions=Index vector (dialog),Index vector (port)  Indices=14,1  OutputSizes=1,1
  Selector9 : Selector  NumberOfDimensions=2  InputPortWidth=3  IndexOptions=Index vector (dialog),Index vector (port)  Indices=15,1  OutputSizes=1,1
  Vector Concatenate : Concatenate  NumInputs=10
  Vector Concatenate1 : Concatenate  NumInputs=10
  Vector Concatenate2 : Concatenate  NumInputs=10
  wheat 1 : Subsystem
  wheat 10 : Subsystem
  wheat 2 : Subsystem
  wheat 3 : Subsystem
  wheat 4 : Subsystem
  wheat 5 : Subsystem
  wheat 6 : Subsystem
  wheat 7 : Subsystem
  wheat 8 : Subsystem
  wheat 9 : Subsystem
  Conn1 : PMIOPort  Side=Left
  wheat height z : Outport
  wheat x : Outport  Port=2
  wheat y : Outport  Port=3
  wires:
  Vector Concatenate/1 -> wheat height z/1
  x force matrix/1 -> Selector1/1, Selector3/1, Selector19/1, Selector17/1, Selector15/1, Selector13/1, Selector11/1, Selector9/1, Selector7/1, Selector5/1
  "column index "/1 -> Selector20/2, Selector19/2, Selector18/2, Selector17/2, Selector16/2, Selector15/2, Selector14/2, Selector13/2, Selector12/2, Selector11/2, Selector10/2, Selector9/2, Selector8/2, Selector7/2, Selector6/2, Selector5/2, Selector4/2, Selector3/2, Selector2/2, Selector1/2
  wheat 1/3(z) -> Vector Concatenate/1
  wheat 9/3(z) -> Vector Concatenate/9
  Selector1/1 -> wheat 1/1(x force)
  Selector13/1 -> wheat 7/1(x force)
  Selector5/1 -> wheat 3/1(x force)
  Selector19/1 -> wheat 10/1(x force)
  Selector16/1 -> wheat 8/2(y force)
  Selector9/1 -> wheat 5/1(x force)
  Selector6/1 -> wheat 3/2(y force)
  Selector15/1 -> wheat 8/1(x force)
  Selector7/1 -> wheat 4/1(x force)
  Selector14/1 -> wheat 7/2(y force)
  Selector11/1 -> wheat 6/1(x force)
  Selector8/1 -> wheat 4/2(y force)
  Selector4/1 -> wheat 2/2(y force)
  Selector20/1 -> wheat 10/2(y force)
  Selector2/1 -> wheat 1/2(y force)
  Selector10/1 -> wheat 5/2(y force)
  wheat 6/3(z) -> Vector Concatenate/6
  Selector12/1 -> wheat 6/2(y force)
  Selector3/1 -> wheat 2/1(x force)
  wheat 10/3(z) -> Vector Concatenate/10
  Selector17/1 -> wheat 9/1(x force)
  y force matrix/1 -> Selector2/1, Selector8/1, Selector20/1, Selector18/1, Selector16/1, Selector14/1, Selector12/1, Selector10/1, Selector6/1, Selector4/1
  Selector18/1 -> wheat 9/2(y force)
  wheat 8/3(z) -> Vector Concatenate/8
  wheat 7/3(z) -> Vector Concatenate/7
  wheat 5/3(z) -> Vector Concatenate/5
  wheat 3/3(z) -> Vector Concatenate/3
  wheat 2/3(z) -> Vector Concatenate/2
  wheat 4/3(z) -> Vector Concatenate/4
  wheat 2/1(x) -> Vector Concatenate1/2
  wheat 3/1(x) -> Vector Concatenate1/3
  wheat 4/1(x) -> Vector Concatenate1/4
  wheat 9/1(x) -> Vector Concatenate1/9
  wheat 10/1(x) -> Vector Concatenate1/10
  Vector Concatenate1/1 -> wheat x/1
  wheat 7/1(x) -> Vector Concatenate1/7
  wheat 5/1(x) -> Vector Concatenate1/5
  wheat 6/1(x) -> Vector Concatenate1/6
  wheat 8/1(x) -> Vector Concatenate1/8
  wheat 1/1(x) -> Vector Concatenate1/1
  wheat 2/2(y) -> Vector Concatenate2/2
  wheat 3/2(y) -> Vector Concatenate2/3
  wheat 4/2(y) -> Vector Concatenate2/4
  wheat 9/2(y) -> Vector Concatenate2/9
  wheat 10/2(y) -> Vector Concatenate2/10
  Vector Concatenate2/1 -> wheat y/1
  wheat 7/2(y) -> Vector Concatenate2/7
  wheat 5/2(y) -> Vector Concatenate2/5
  wheat 6/2(y) -> Vector Concatenate2/6
  wheat 8/2(y) -> Vector Concatenate2/8
  wheat 1/2(y) -> Vector Concatenate2/1
  connections:
  wheat 5/LConn1 -- Rigid Transform4/RConn1
  wheat 3/LConn1 -- Rigid Transform2/RConn1
  wheat 4/LConn1 -- Rigid Transform3/RConn1
  Rigid Transform5/RConn1 -- wheat 6/LConn1
  Rigid Transform9/RConn1 -- wheat 9/LConn1
  wheat 8/LConn1 -- Rigid Transform8/RConn1
  wheat 7/LConn1 -- Rigid Transform6/RConn1
  Rigid Transform10/RConn1 -- wheat 10/LConn1
  wheat 2/LConn1 -- Rigid Transform1/RConn1
  Rigid Transform10/LConn1 -- Rigid Transform9/LConn1 -- Rigid Transform8/LConn1 -- Rigid Transform6/LConn1 -- Rigid Transform5/LConn1 -- Rigid Transform4/LConn1 -- Rigid Transform3/LConn1 -- Rigid Transform2/LConn1 -- Rigid Transform1/LConn1 -- Conn1/RConn1 -- wheat 1/LConn1

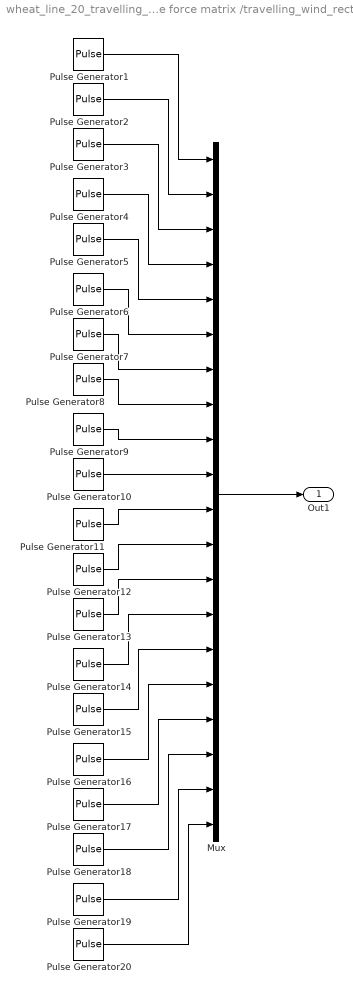
== system wheat_line_20_travelling_wind_2019b/calculate force matrix /travelling_wind_rectangle ==
  Mux : Mux  Inputs=20
  Pulse Generator1 : DiscretePulseGenerator  PulseType=Time based  Amplitude=wind_amplitude  Period=1/wind_frequency  PulseWidth=50  PhaseDelay=1/wind_phase_cycle*1
  Pulse Generator10 : DiscretePulseGenerator  PulseType=Time based  Amplitude=wind_amplitude  Period=1/wind_frequency  PulseWidth=50  PhaseDelay=1/wind_phase_cycle*10
  Pulse Generator11 : DiscretePulseGenerator  PulseType=Time based  Amplitude=wind_amplitude  Period=1/wind_frequency  PulseWidth=50  PhaseDelay=1/wind_phase_cycle*11
  Pulse Generator12 : DiscretePulseGenerator  PulseType=Time based  Amplitude=wind_amplitude  Period=1/wind_frequency  PulseWidth=50  PhaseDelay=1/wind_phase_cycle*12
  Pulse Generator13 : DiscretePulseGenerator  PulseType=Time based  Amplitude=wind_amplitude  Period=1/wind_frequency  PulseWidth=50  PhaseDelay=1/wind_phase_cycle*13
  Pulse Generator14 : DiscretePulseGenerator  PulseType=Time based  Amplitude=wind_amplitude  Period=1/wind_frequency  PulseWidth=50  PhaseDelay=1/wind_phase_cycle*14
  Pulse Generator15 : DiscretePulseGenerator  PulseType=Time based  Amplitude=wind_amplitude  Period=1/wind_frequency  PulseWidth=50  PhaseDelay=1/wind_phase_cycle*15
  Pulse Generator16 : DiscretePulseGenerator  PulseType=Time based  Amplitude=wind_amplitude  Period=1/wind_frequency  PulseWidth=50  PhaseDelay=1/wind_phase_cycle*16
  Pulse Generator17 : DiscretePulseGenerator  PulseType=Time based  Amplitude=wind_amplitude  Period=1/wind_frequency  PulseWidth=50  PhaseDelay=1/wind_phase_cycle*17
  Pulse Generator18 : DiscretePulseGenerator  PulseType=Time based  Amplitude=wind_amplitude  Period=1/wind_frequency  PulseWidth=50  PhaseDelay=1/wind_phase_cycle*18
  Pulse Generator19 : DiscretePulseGenerator  PulseType=Time based  Amplitude=wind_amplitude  Period=1/wind_frequency  PulseWidth=50  PhaseDelay=1/wind_phase_cycle*19
  Pulse Generator2 : DiscretePulseGenerator  PulseType=Time based  Amplitude=wind_amplitude  Period=1/wind_frequency  PulseWidth=50  PhaseDelay=1/wind_phase_cycle*2
  Pulse Generator20 : DiscretePulseGenerator  PulseType=Time based  Amplitude=wind_amplitude  Period=1/wind_frequency  PulseWidth=50  PhaseDelay=1/wind_phase_cycle*20
  Pulse Generator3 : DiscretePulseGenerator  PulseType=Time based  Amplitude=wind_amplitude  Period=1/wind_frequency  PulseWidth=50  PhaseDelay=1/wind_phase_cycle*3
  Pulse Generator4 : DiscretePulseGenerator  PulseType=Time based  Amplitude=wind_amplitude  Period=1/wind_frequency  PulseWidth=50  PhaseDelay=1/wind_phase_cycle*4
  Pulse Generator5 : DiscretePulseGenerator  PulseType=Time based  Amplitude=wind_amplitude  Period=1/wind_frequency  PulseWidth=50  PhaseDelay=1/wind_phase_cycle*5
  Pulse Generator6 : DiscretePulseGenerator  PulseType=Time based  Amplitude=wind_amplitude  Period=1/wind_frequency  PulseWidth=50  PhaseDelay=1/wind_phase_cycle*6
  Pulse Generator7 : DiscretePulseGenerator  PulseType=Time based  Amplitude=wind_amplitude  Period=1/wind_frequency  PulseWidth=50  PhaseDelay=1/wind_phase_cycle*7
  Pulse Generator8 : DiscretePulseGenerator  PulseType=Time based  Amplitude=wind_amplitude  Period=1/wind_frequency  PulseWidth=50  PhaseDelay=1/wind_phase_cycle*8
  Pulse Generator9 : DiscretePulseGenerator  PulseType=Time based  Amplitude=wind_amplitude  Period=1/wind_frequency  PulseWidth=50  PhaseDelay=1/wind_phase_cycle*9
  Out1 : Outport
  wires:
  Pulse Generator17/1 -> Mux/17
  Pulse Generator18/1 -> Mux/18
  Pulse Generator6/1 -> Mux/6
  Pulse Generator19/1 -> Mux/19
  Pulse Generator16/1 -> Mux/16
  Pulse Generator13/1 -> Mux/13
  Pulse Generator20/1 -> Mux/20
  Pulse Generator14/1 -> Mux/14
  Pulse Generator12/1 -> Mux/12
  Pulse Generator15/1 -> Mux/15
  Pulse Generator11/1 -> Mux/11
  Pulse Generator10/1 -> Mux/10
  Pulse Generator9/1 -> Mux/9
  Pulse Generator8/1 -> Mux/8
  Pulse Generator7/1 -> Mux/7
  Pulse Generator5/1 -> Mux/5
  Pulse Generator4/1 -> Mux/4
  Pulse Generator3/1 -> Mux/3
  Pulse Generator2/1 -> Mux/2
  Pulse Generator1/1 -> Mux/1
  Mux/1 -> Out1/1

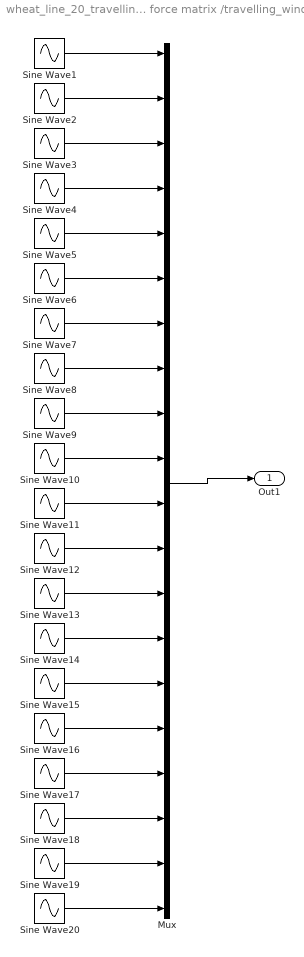
== system wheat_line_20_travelling_wind_2019b/calculate force matrix /travelling_wind_sine ==
  Mux : Mux  Inputs=20
  Sine Wave1 : Sin  Amplitude=wind_amplitude  Frequency=wind_frequency  Phase=2*pi/wind_phase_cycle*1  SampleTime=0
  Sine Wave10 : Sin  Amplitude=wind_amplitude  Frequency=wind_frequency  Phase=2*pi/wind_phase_cycle*10  SampleTime=0
  Sine Wave11 : Sin  Amplitude=wind_amplitude  Frequency=wind_frequency  Phase=2*pi/wind_phase_cycle*11  SampleTime=0
  Sine Wave12 : Sin  Amplitude=wind_amplitude  Frequency=wind_frequency  Phase=2*pi/wind_phase_cycle*12  SampleTime=0
  Sine Wave13 : Sin  Amplitude=wind_amplitude  Frequency=wind_frequency  Phase=2*pi/wind_phase_cycle*13  SampleTime=0
  Sine Wave14 : Sin  Amplitude=wind_amplitude  Frequency=wind_frequency  Phase=2*pi/wind_phase_cycle*14  SampleTime=0
  Sine Wave15 : Sin  Amplitude=wind_amplitude  Frequency=wind_frequency  Phase=2*pi/wind_phase_cycle*15  SampleTime=0
  Sine Wave16 : Sin  Amplitude=wind_amplitude  Frequency=wind_frequency  Phase=2*pi/wind_phase_cycle*16  SampleTime=0
  Sine Wave17 : Sin  Amplitude=wind_amplitude  Frequency=wind_frequency  Phase=2*pi/wind_phase_cycle*17  SampleTime=0
  Sine Wave18 : Sin  Amplitude=wind_amplitude  Frequency=wind_frequency  Phase=2*pi/wind_phase_cycle*18  SampleTime=0
  Sine Wave19 : Sin  Amplitude=wind_amplitude  Frequency=wind_frequency  Phase=2*pi/wind_phase_cycle*19  SampleTime=0
  Sine Wave2 : Sin  Amplitude=wind_amplitude  Frequency=wind_frequency  Phase=2*pi/wind_phase_cycle*2  SampleTime=0
  Sine Wave20 : Sin  Amplitude=wind_amplitude  Frequency=wind_frequency  Phase=2*pi/wind_phase_cycle*20  SampleTime=0
  Sine Wave3 : Sin  Amplitude=wind_amplitude  Frequency=wind_frequency  Phase=2*pi/wind_phase_cycle*3  SampleTime=0
  Sine Wave4 : Sin  Amplitude=wind_amplitude  Frequency=wind_frequency  Phase=2*pi/wind_phase_cycle*4  SampleTime=0
  Sine Wave5 : Sin  Amplitude=wind_amplitude  Frequency=wind_frequency  Phase=2*pi/wind_phase_cycle*5  SampleTime=0
  Sine Wave6 : Sin  Amplitude=wind_amplitude  Frequency=wind_frequency  Phase=2*pi/wind_phase_cycle*6  SampleTime=0
  Sine Wave7 : Sin  Amplitude=wind_amplitude  Frequency=wind_frequency  Phase=2*pi/wind_phase_cycle*7  SampleTime=0
  Sine Wave8 : Sin  Amplitude=wind_amplitude  Frequency=wind_frequency  Phase=2*pi/wind_phase_cycle*8  SampleTime=0
  Sine Wave9 : Sin  Amplitude=wind_amplitude  Frequency=wind_frequency  Phase=2*pi/wind_phase_cycle*9  SampleTime=0
  Out1 : Outport
  wires:
  Sine Wave6/1 -> Mux/6
  Sine Wave13/1 -> Mux/13
  Sine Wave20/1 -> Mux/20
  Sine Wave8/1 -> Mux/8
  Sine Wave1/1 -> Mux/1
  Sine Wave10/1 -> Mux/10
  Sine Wave3/1 -> Mux/3
  Sine Wave9/1 -> Mux/9
  Sine Wave2/1 -> Mux/2
  Sine Wave7/1 -> Mux/7
  Sine Wave5/1 -> Mux/5
  Sine Wave12/1 -> Mux/12
  Sine Wave4/1 -> Mux/4
  Sine Wave11/1 -> Mux/11
  Sine Wave16/1 -> Mux/16
  Sine Wave17/1 -> Mux/17
  Sine Wave15/1 -> Mux/15
  Sine Wave14/1 -> Mux/14
  Sine Wave19/1 -> Mux/19
  Sine Wave18/1 -> Mux/18
  Mux/1 -> Out1/1
